simulink model "Aearial_Inspection_UAV_Simulation"  (R2023a)
settings: Solver=daessc  StartTime=0.0  StopTime=tf  MaxStep=0.1  MinStep=1e-30  RelTol=1e-4
values from neighbouring files (symbols this model uses):
  arm_start = 0    [InitScript.m]
  X = T*[x0;y0]    [line2circle.m]
undefined symbols (not defined in the file or in its folder): arm_end, DiscIntNeverNeededParam, F, is_gust_active, Light, MIL, Mode, Motor_data, params, Robotic_Arm_ASM_DataFile, Sensor_err, servo_specs, simple_env, stepper, Tm, wind_speed, xStack1, xStack2, Y, Z
libraries: sm_lib x399, nesl_utility x78, simulink x25, dspsrcs4 x16, simulink_extras x8, sharedtransform x7, aerolibwind2 x2, sharedutil x1
(part 4 of 12)

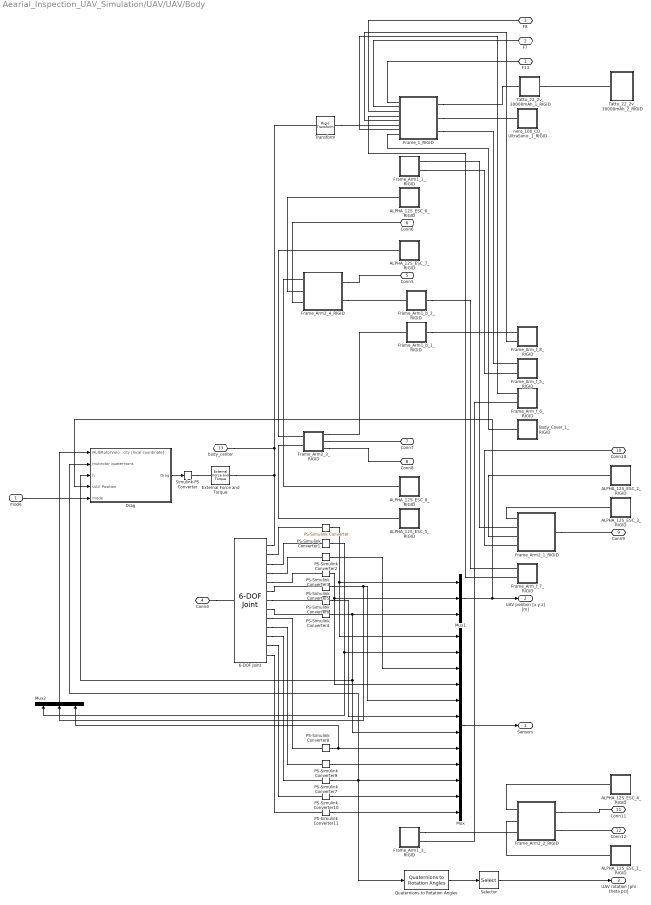
== system Aearial_Inspection_UAV_Simulation/UAV/UAV/Body ==
  mode : Inport
  " " : nesl_utility/PS-Simulink Converter  PhysicalDomain=network_engine_domain  SubClassName=ps_output  LeftPortType=input  RightPortType=output  PseudoPeriodic=off  Frequencies=[]  VectorFormat=1-D array  Unit=m  AffineConversion=off
  6-DOF Joint : sm_lib/Joints/6-DOF Joint  JointMode=Normal  SenseConstraintForce=off  SenseConstraintForceX=off  SenseConstraintForceY=off  SenseConstraintForceZ=off  SenseConstraintTorque=off  SenseConstraintTorqueX=off  SenseConstraintTorqueY=off  SenseConstraintTorqueZ=off  SenseTotalForce=off  SenseTotalForceX=off  SenseTotalForceY=off  SenseTotalForceZ=off  SenseTotalTorque=off  SenseTotalTorqueX=off  SenseTotalTorqueY=off  SenseTotalTorqueZ=off  CompositeWrenchDir=FollowerOnBase  CompositeWrenchFrame=BaseFrame  PxEquilibriumPosition=0  PxEquilibriumPositionUnits=m  PxSpringStiffness=0  PxSpringStiffnessUnits=N/m  PxDampingCoefficient=0  PxDampingCoefficientUnits=N/(m/s)  PxTorqueActuationMode=NoTorque  PxMotionActuationMode=ComputedMotion  PxSensePosition=on  PxSenseVelocity=on  PxSenseAcceleration=on  PxSenseTorqueForce=off  PxSenseLowerLimitTorqueForce=off  PxSenseUpperLimitTorqueForce=off  PxLowerLimitSpecify=off  PxLowerLimitBound=-1  PxLowerLimitBoundUnits=m  PxLowerLimitStiffness=1e6  PxLowerLimitStiffnessUnits=N/m  PxLowerLimitDamping=1e3  PxLowerLimitDampingUnits=N/(m/s)  PxLowerLimitTransitionRegionWidth=1e-4  PxLowerLimitTransitionRegionWidthUnits=m  PxUpperLimitSpecify=off  PxUpperLimitBound=1  PxUpperLimitBoundUnits=m  PxUpperLimitStiffness=1e6  PxUpperLimitStiffnessUnits=N/m  PxUpperLimitDamping=1e3  PxUpperLimitDampingUnits=N/(m/s)  PxUpperLimitTransitionRegionWidth=1e-4  PxUpperLimitTransitionRegionWidthUnits=m  PxPositionTargetSpecify=on  PxPositionTargetPriority=High  PxPositionTargetValue=params.pos0(1)  PxPositionTargetValueUnits=m  PxVelocityTargetSpecify=on  PxVelocityTargetPriority=High  PxVelocityTargetValue=params.vel0(1)  PxVelocityTargetValueUnits=m/s  PyEquilibriumPosition=0  PyEquilibriumPositionUnits=m  PySpringStiffness=0  PySpringStiffnessUnits=N/m  PyDampingCoefficient=0  PyDampingCoefficientUnits=N/(m/s)  PyTorqueActuationMode=NoTorque  PyMotionActuationMode=ComputedMotion  PySensePosition=on  PySenseVelocity=on  PySenseAcceleration=on  PySenseTorqueForce=off  PySenseLowerLimitTorqueForce=off  PySenseUpperLimitTorqueForce=off  PyLowerLimitSpecify=off  PyLowerLimitBound=-1  PyLowerLimitBoundUnits=m  PyLowerLimitStiffness=1e6  PyLowerLimitStiffnessUnits=N/m  PyLowerLimitDamping=1e3  PyLowerLimitDampingUnits=N/(m/s)  PyLowerLimitTransitionRegionWidth=1e-4  PyLowerLimitTransitionRegionWidthUnits=m  PyUpperLimitSpecify=off  PyUpperLimitBound=1  PyUpperLimitBoundUnits=m  PyUpperLimitStiffness=1e6  PyUpperLimitStiffnessUnits=N/m  PyUpperLimitDamping=1e3  PyUpperLimitDampingUnits=N/(m/s)  PyUpperLimitTransitionRegionWidth=1e-4  PyUpperLimitTransitionRegionWidthUnits=m  PyPositionTargetSpecify=on  PyPositionTargetPriority=High  PyPositionTargetValue=params.pos0(2)  PyPositionTargetValueUnits=m  PyVelocityTargetSpecify=on  PyVelocityTargetPriority=High  PyVelocityTargetValue=params.vel0(2)  PyVelocityTargetValueUnits=m/s  PzEquilibriumPosition=0  PzEquilibriumPositionUnits=m  PzSpringStiffness=0  PzSpringStiffnessUnits=N/m  PzDampingCoefficient=0  PzDampingCoefficientUnits=N/(m/s)  PzTorqueActuationMode=NoTorque  PzMotionActuationMode=ComputedMotion  PzSensePosition=on  PzSenseVelocity=on  PzSenseAcceleration=on  PzSenseTorqueForce=off  PzSenseLowerLimitTorqueForce=off  PzSenseUpperLimitTorqueForce=off  PzLowerLimitSpecify=off  PzLowerLimitBound=-1  PzLowerLimitBoundUnits=m  PzLowerLimitStiffness=1e6  PzLowerLimitStiffnessUnits=N/m  PzLowerLimitDamping=1e3  PzLowerLimitDampingUnits=N/(m/s)  PzLowerLimitTransitionRegionWidth=1e-4  PzLowerLimitTransitionRegionWidthUnits=m  PzUpperLimitSpecify=off  PzUpperLimitBound=1  PzUpperLimitBoundUnits=m  PzUpperLimitStiffness=1e6  PzUpperLimitStiffnessUnits=N/m  PzUpperLimitDamping=1e3  PzUpperLimitDampingUnits=N/(m/s)  PzUpperLimitTransitionRegionWidth=1e-4  PzUpperLimitTransitionRegionWidthUnits=m  PzPositionTargetSpecify=on  PzPositionTargetPriority=High  PzPositionTargetValue=params.pos0(3)  PzPositionTargetValueUnits=m  PzVelocityTargetSpecify=on  PzVelocityTargetPriority=High  PzVelocityTargetValue=params.vel0(3)  PzVelocityTargetValueUnits=m/s  SphEqPosRotationMethod=None  SphEqPosRotationAngleUnits=deg  SphEqPosRotationStandardAxis=+Z  SphEqPosRotationAngle=0.0  SphEqPosRotationArbitraryAxis=[0 0 1]  SphEqPosFollAlignAxisA=+X  SphEqPosBaseAlignAxisA=+Y  SphEqPosFollAlignAxisB=+Y  SphEqPosBaseAlignAxisB=+Z  SphEqPosRotationSequenceAxes=FollowerAxes  SphEqPosRotationSequence=XYX  SphEqPosRotationSequenceAngles=[0 0 0]  SphEqPosRotationSequenceAnglesUnits=deg  SphEqPosRotationMatrix=[1 0 0; 0 1 0; 0 0 1]  SphEqPosQuaternion=[1 0 0 0]  SphSpringStiffness=0  SphSpringStiffnessUnits=N*m/deg  SphDampingCoefficient=0  SphDampingCoefficientUnits=N*m/(deg/s)  SphActuateTorqueX=off  SphActuateTorqueY=off  SphActuateTorqueZ=off  SphActuateTorque=off  SphTorqueActuationMode=NoTorque  SphMotionActuationMode=ComputedMotion  SphActuationFrame=BaseFrame  SphSensePosition=on  SphSenseVelocityX=off  SphSenseVelocityY=off  SphSenseVelocityZ=off  SphSenseVelocity=on  SphSenseAccelerationX=off  SphSenseAccelerationY=off  SphSenseAccelerationZ=off  SphSenseAcceleration=on  SphSenseTorqueX=off  SphSenseTorqueY=off  SphSenseTorqueZ=off  SphSenseTorqueForce=off  SphSenseLowerLimitTorqueMag=off  SphSenseUpperLimitTorqueMag=off  SphSensingFrame=FollowerFrame  SphLowerLimitSpecify=off  SphLowerLimitBound=15  SphLowerLimitBoundUnits=deg  SphLowerLimitStiffness=1e4  SphLowerLimitStiffnessUnits=N*m/deg  SphLowerLimitDamping=10  SphLowerLimitDampingUnits=N*m/(deg/s)  SphLowerLimitTransitionRegionWidth=0.1  SphLowerLimitTransitionRegionWidthUnits=deg  SphUpperLimitSpecify=off  SphUpperLimitBound=45  SphUpperLimitBoundUnits=deg  SphUpperLimitStiffness=1e4  SphUpperLimitStiffnessUnits=N*m/deg  SphUpperLimitDamping=10  SphUpperLimitDampingUnits=N*m/(deg/s)  SphUpperLimitTransitionRegionWidth=0.1  SphUpperLimitTransitionRegionWidthUnits=deg  SphPositionTargetRotationMethod=RotationSequence  SphPositionTargetRotationAngleUnits=deg  SphPositionTargetRotationStandardAxis=+Z  SphPositionTargetRotationAngle=0.0  SphPositionTargetRotationArbitraryAxis=[0 0 1]  SphPositionTargetFollAlignAxisA=+X  SphPositionTargetBaseAlignAxisA=+Y  SphPositionTargetFollAlignAxisB=+Y  SphPositionTargetBaseAlignAxisB=+Z  SphPositionTargetRotationSequenceAxes=FollowerAxes  SphPositionTargetRotationSequence=XYZ  SphPositionTargetRotationSequenceAngles=params.Eul0  SphPositionTargetRotationSequenceAnglesUnits=deg  SphPositionTargetRotationMatrix=[1 0 0; 0 1 0; 0 0 1]  SphPositionTargetQuaternion=[1 0 0 0]  SphPositionTargetSpecify=on  SphPositionTargetPriority=High  SphVelocityTargetValue=params.Avel0  SphVelocityTargetValueUnits=deg/s  SphVelocityTargetSpecify=on  SphVelocityTargetPriority=High  SphVelocityTargetInFollowerFrame=on
  ALPHA_12S_ESC_1_RIGID : Subsystem
  ALPHA_12S_ESC_2_RIGID : Subsystem
  ALPHA_12S_ESC_3_RIGID : Subsystem
  ALPHA_12S_ESC_4_RIGID : Subsystem
  ALPHA_12S_ESC_5_RIGID : Subsystem
  ALPHA_12S_ESC_6_RIGID : Subsystem
  ALPHA_12S_ESC_7_RIGID : Subsystem
  ALPHA_12S_ESC_8_RIGID : Subsystem
  Body_Cover_1_RIGID : Subsystem
  Drag : Subsystem
  External Force and Torque : sm_lib/Forces and Torques/External Force and Torque  ForceResolutionFrame=AttachedFrame  EnableForceX=off  EnableForceY=off  EnableForceZ=off  EnableForce=on  TorqueResolutionFrame=AttachedFrame  EnableTorqueX=off  EnableTorqueY=off  EnableTorqueZ=off  EnableTorque=off
  Frame_1_RIGID : Subsystem
  Frame_Arm1_1_RIGID : Subsystem
  Frame_Arm1_3_RIGID : Subsystem
  Frame_Arm1_b_1_RIGID : Subsystem
  Frame_Arm1_b_2_RIGID : Subsystem
  Frame_Arm2_1_RIGID : Subsystem
  Frame_Arm2_2_RIGID : Subsystem
  Frame_Arm2_3_RIGID : Subsystem
  Frame_Arm2_4_RIGID : Subsystem
  Frame_Arm_f_5_RIGID : Subsystem
  Frame_Arm_f_6_RIGID : Subsystem
  Frame_Arm_f_7_RIGID : Subsystem
  Frame_Arm_f_8_RIGID : Subsystem
  Mux : Mux  Inputs=12
  Mux1 : Mux  Inputs=3
  Mux2 : Mux  Inputs=3
  PS-Simulink Converter1 : nesl_utility/PS-Simulink Converter  PhysicalDomain=network_engine_domain  SubClassName=ps_output  LeftPortType=input  RightPortType=output  PseudoPeriodic=off  Frequencies=[]  VectorFormat=1-D array  Unit=m/s  AffineConversion=off
  PS-Simulink Converter10 : nesl_utility/PS-Simulink Converter  PhysicalDomain=network_engine_domain  SubClassName=ps_output  LeftPortType=input  RightPortType=output  PseudoPeriodic=off  Frequencies=[]  VectorFormat=1-D array  Unit=rad/s  AffineConversion=off
  PS-Simulink Converter11 : nesl_utility/PS-Simulink Converter  PhysicalDomain=network_engine_domain  SubClassName=ps_output  LeftPortType=input  RightPortType=output  PseudoPeriodic=off  Frequencies=[]  VectorFormat=1-D array  Unit=rad/s^2  AffineConversion=off
  PS-Simulink Converter2 : nesl_utility/PS-Simulink Converter  PhysicalDomain=network_engine_domain  SubClassName=ps_output  LeftPortType=input  RightPortType=output  PseudoPeriodic=off  Frequencies=[]  VectorFormat=1-D array  Unit=m/s^2  AffineConversion=off
  PS-Simulink Converter3 : nesl_utility/PS-Simulink Converter  PhysicalDomain=network_engine_domain  SubClassName=ps_output  LeftPortType=input  RightPortType=output  PseudoPeriodic=off  Frequencies=[]  VectorFormat=1-D array  Unit=m  AffineConversion=off
  PS-Simulink Converter4 : nesl_utility/PS-Simulink Converter  PhysicalDomain=network_engine_domain  SubClassName=ps_output  LeftPortType=input  RightPortType=output  PseudoPeriodic=off  Frequencies=[]  VectorFormat=1-D array  Unit=m  AffineConversion=off
  PS-Simulink Converter5 : nesl_utility/PS-Simulink Converter  PhysicalDomain=network_engine_domain  SubClassName=ps_output  LeftPortType=input  RightPortType=output  PseudoPeriodic=off  Frequencies=[]  VectorFormat=1-D array  Unit=m/s  AffineConversion=off
  PS-Simulink Converter6 : nesl_utility/PS-Simulink Converter  PhysicalDomain=network_engine_domain  SubClassName=ps_output  LeftPortType=input  RightPortType=output  PseudoPeriodic=off  Frequencies=[]  VectorFormat=1-D array  Unit=m/s^2  AffineConversion=off
  PS-Simulink Converter7 : nesl_utility/PS-Simulink Converter  PhysicalDomain=network_engine_domain  SubClassName=ps_output  LeftPortType=input  RightPortType=output  PseudoPeriodic=off  Frequencies=[]  VectorFormat=1-D array  Unit=inherit  AffineConversion=off
  PS-Simulink Converter8 : nesl_utility/PS-Simulink Converter  PhysicalDomain=network_engine_domain  SubClassName=ps_output  LeftPortType=input  RightPortType=output  PseudoPeriodic=off  Frequencies=[]  VectorFormat=1-D array  Unit=m/s  AffineConversion=off
  PS-Simulink Converter9 : nesl_utility/PS-Simulink Converter  PhysicalDomain=network_engine_domain  SubClassName=ps_output  LeftPortType=input  RightPortType=output  PseudoPeriodic=off  Frequencies=[]  VectorFormat=1-D array  Unit=m/s^2  AffineConversion=off
  Quaternions to Rotation Angles : sharedtransform/Quaternions to Rotation Angles  rotationOrder=ZYX  aMode=aMode
  Selector : Selector  InputPortWidth=3  IndexOptions=Index vector (dialog)  Indices=[3 2 1]  OutputSizes=1
  Simulink-PS Converter : nesl_utility/Simulink-PS Converter  PhysicalDomain=network_engine_domain  SubClassName=ps_input  LeftPortType=input  RightPortType=output  PseudoPeriodic=off  Frequencies=[]  NoiseDistribution=none  NoiseParameters=[]  Unit=N  AffineConversion=off  FilteringAndDerivatives=provide  SimscapeFilterOrder=1  InputFilterTimeConstant=0.001  UdotUserProvided=0
  Tattu_22_2v_30000mAh_1_RIGID : Subsystem
  Tattu_22_2v_30000mAh_2_RIGID : Subsystem
  Transform : sm_lib/Frames and Transforms/Rigid Transform  TranslationMethod=Cartesian  TranslationStandardOffset=0  TranslationStandardOffsetUnits=mm  TranslationStandardAxis=+Z  TranslationCartesianOffset=[0.2 0 0]  TranslationCartesianOffsetUnits=mm  TranslationROffset=0  TranslationROffsetUnits=m  TranslationZOffset=0  TranslationZOffsetUnits=m  TranslationThetaOffset=0  TranslationThetaOffsetUnits=deg  RotationMethod=AlignedAxes  RotationAngleUnits=rad  RotationStandardAxis=+Z  RotationAngle=smiData.RigidTransform(347).angle  RotationArbitraryAxis=smiData.RigidTransform(347).axis  FollAlignAxisA=+X  BaseAlignAxisA=+Y  FollAlignAxisB=+Y  BaseAlignAxisB=-Z  RotationSequenceAxes=FollowerAxes  RotationSequence=XYX  RotationSequenceAngles=[0 0 0]  RotationSequenceAnglesUnits=deg  RotationMatrix=[1 0 0; 0 1 0; 0 0 1]  Quaternion=[1 0 0 0]
  nero_100_CD_UltraSonic_1_RIGID : Subsystem
  F13 : PMIOPort  Side=Left
  F7 : PMIOPort  Port=2  Side=Left
  F8 : PMIOPort  Port=3  Side=Left
  Conn4 : PMIOPort  Port=4  Side=Left
  Conn5 : PMIOPort  Port=5  Side=Right
  Conn6 : PMIOPort  Port=6  Side=Right
  Conn7 : PMIOPort  Port=7  Side=Right
  Conn8 : PMIOPort  Port=8  Side=Right
  Conn9 : PMIOPort  Port=9  Side=Right
  Conn10 : PMIOPort  Port=10  Side=Right
  Conn11 : PMIOPort  Port=11  Side=Right
  Conn12 : PMIOPort  Port=12  Side=Right
  body_center : PMIOPort  Port=13  Side=Left
  Sensors : Outport
  UAV position [x y z] [m] : Outport  Port=2
  UAV rotation [phi theta psi] : Outport  Port=3
  wires:
  PS-Simulink Converter8/1 -> Mux2/3, Mux/8
  Mux/1 -> Sensors/1
  PS-Simulink Converter10/1 -> Mux/11
  Quaternions to Rotation Angles/1 -> Selector/1
  Mux1/1 -> Drag/4(UAV Position), UAV position [x y z] [m]/1
  PS-Simulink Converter11/1 -> Mux/12
  PS-Simulink Converter9/1 -> Mux/9
  PS-Simulink Converter6/1 -> Mux/6
  PS-Simulink Converter5/1 -> Mux2/2, Mux/5
  PS-Simulink Converter2/1 -> Mux/3
  PS-Simulink Converter1/1 -> Mux2/1, Mux/2
  PS-Simulink Converter7/1 -> Quaternions to Rotation Angles/1, Drag/2(mutirotor quaternions), Mux/10
  PS-Simulink Converter4/1 -> Drag/3(h), Mux/7, Mux1/3
  PS-Simulink Converter3/1 -> Mux1/2, Mux/4
  " "/1 -> Mux1/1, Mux/1
  Mux2/1 -> Drag/1(MultiRotorVelocity [local coordinate])
  Drag/1(Drag) -> Simulink-PS Converter/1
  mode/1 -> Drag/5(mode)
  Selector/1 -> UAV rotation [phi theta psi]/1
  connections:
  6-DOF Joint/RConn11 -- PS-Simulink Converter7/LConn1
  Transform/RConn1 -- Frame_1_RIGID/LConn6
  ALPHA_12S_ESC_5_RIGID/LConn1 -- Frame_Arm2_3_RIGID/LConn2
  Frame_1_RIGID/LConn3 -- F8/RConn1
  6-DOF Joint/RConn6 -- PS-Simulink Converter5/LConn1
  Frame_Arm2_2_RIGID/RConn2 -- Conn12/RConn1
  ALPHA_12S_ESC_3_RIGID/LConn1 -- Frame_Arm2_1_RIGID/LConn1
  Frame_1_RIGID/RConn2 -- nero_100_CD_UltraSonic_1_RIGID/LConn1
  6-DOF Joint/RConn13 -- PS-Simulink Converter11/LConn1
  ALPHA_12S_ESC_6_RIGID/LConn1 -- Frame_Arm2_4_RIGID/LConn2
  Frame_1_RIGID/RConn1 -- Tattu_22_2v_30000mAh_1_RIGID/LConn1
  6-DOF Joint/RConn12 -- PS-Simulink Converter10/LConn1
  Frame_1_RIGID/LConn7 -- Frame_Arm_f_6_RIGID/LConn1
  6-DOF Joint/RConn10 -- PS-Simulink Converter9/LConn1
  6-DOF Joint/RConn9 -- PS-Simulink Converter8/LConn1
  Frame_1_RIGID/LConn4 -- Frame_Arm_f_7_RIGID/LConn2
  6-DOF Joint/RConn7 -- PS-Simulink Converter6/LConn1
  Frame_1_RIGID/LConn5 -- Frame_Arm_f_8_RIGID/LConn2
  6-DOF Joint/RConn8 -- PS-Simulink Converter4/LConn1
  6-DOF Joint/RConn5 -- PS-Simulink Converter3/LConn1
  6-DOF Joint/RConn4 -- PS-Simulink Converter2/LConn1
  6-DOF Joint/RConn3 -- PS-Simulink Converter1/LConn1
  6-DOF Joint/RConn2 -- " "/LConn1
  6-DOF Joint/RConn1 -- External Force and Torque/RConn1 -- body_center/RConn1 -- Transform/LConn1
  ALPHA_12S_ESC_4_RIGID/LConn1 -- Frame_Arm2_2_RIGID/LConn1
  F13/RConn1 -- Frame_1_RIGID/LConn1
  Conn4/RConn1 -- 6-DOF Joint/LConn1
  Frame_Arm1_3_RIGID/RConn2 -- Frame_Arm_f_6_RIGID/LConn2
  Frame_Arm2_1_RIGID/LConn4 -- Conn10/RConn1
  Tattu_22_2v_30000mAh_1_RIGID/RConn1 -- Tattu_22_2v_30000mAh_2_RIGID/LConn1
  F7/RConn1 -- Frame_1_RIGID/LConn2
  Conn6/RConn1 -- Frame_Arm2_4_RIGID/LConn3
  Frame_Arm1_b_2_RIGID/RConn1 -- Frame_Arm_f_7_RIGID/LConn1
  ALPHA_12S_ESC_2_RIGID/LConn1 -- Frame_Arm2_1_RIGID/LConn3
  Frame_Arm2_2_RIGID/RConn1 -- Conn11/RConn1
  Frame_Arm1_1_RIGID/RConn2 -- Frame_Arm_f_5_RIGID/LConn2
  Frame_1_RIGID/RConn3 -- Frame_Arm_f_5_RIGID/LConn1
  ALPHA_12S_ESC_1_RIGID/LConn1 -- Frame_Arm2_2_RIGID/LConn2
  ALPHA_12S_ESC_8_RIGID/LConn1 -- Frame_Arm2_4_RIGID/LConn1
  Body_Cover_1_RIGID/LConn1 -- Frame_1_RIGID/LConn8
  Frame_Arm2_3_RIGID/RConn1 -- Frame_Arm1_b_1_RIGID/LConn1
  Frame_Arm2_1_RIGID/RConn1 -- Conn9/RConn1
  Frame_Arm2_4_RIGID/RConn2 -- Frame_Arm1_b_2_RIGID/LConn1
  Frame_Arm2_3_RIGID/RConn3 -- Conn8/RConn1
  Frame_Arm1_3_RIGID/RConn1 -- Frame_Arm2_2_RIGID/LConn3
  Frame_Arm2_4_RIGID/RConn1 -- Conn5/RConn1
  Frame_Arm2_3_RIGID/RConn2 -- Conn7/RConn1
  ALPHA_12S_ESC_7_RIGID/LConn1 -- Frame_Arm2_3_RIGID/LConn1
  Frame_Arm1_b_1_RIGID/RConn1 -- Frame_Arm_f_8_RIGID/LConn1
  Frame_Arm1_1_RIGID/RConn1 -- Frame_Arm2_1_RIGID/LConn2
  Simulink-PS Converter/RConn1 -- External Force and Torque/LConn1

== system Aearial_Inspection_UAV_Simulation/UAV/UAV/Device ==
  Device_1_RIGID : Subsystem
  Device_Box_1_RIGID : Subsystem
  F : PMIOPort  Side=Left
  connections:
  Device_1_RIGID/LConn1 -- Device_Box_1_RIGID/LConn1
  Device_Box_1_RIGID/LConn2 -- F/RConn1

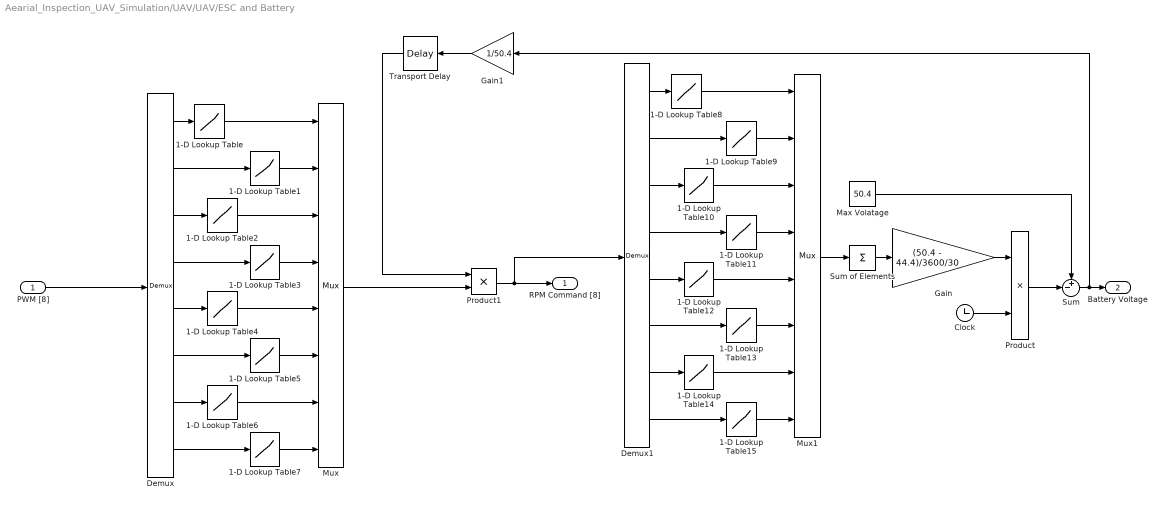
== system Aearial_Inspection_UAV_Simulation/UAV/UAV/ESC and Battery ==
  PWM [8] : Inport
  1-D Lookup Table{,1..7} (8 alike) : Lookup_n-D  NumberOfTableDimensions=1  BreakpointsForDimension1=[0;Motor_data.Throttle]  Table=[0;Motor_data.RPM]  InternalRulePriority=Speed  RndMeth=Simplest
  1-D Lookup Table{8..15} (8 alike) : Lookup_n-D  NumberOfTableDimensions=1  BreakpointsForDimension1=[0;Motor_data.RPM]  Table=[0;Motor_data.Current]  InterpMethod=Cubic spline  ExtrapMethod=Cubic spline  InternalRulePriority=Speed  RndMeth=Simplest
  Clock : Clock
  Demux : Demux  Outputs=8
  Demux1 : Demux  Outputs=8
  Gain : Gain  Gain=(50.4 - 44.4)/3600/30
  Gain1 : Gain  Gain=1/50.4
  Max Volatage : Constant  Value=50.4
  Mux : Mux  Inputs=8
  Mux1 : Mux  Inputs=8
  Product : Product
  Product1 : Product
  Sum : Sum  Inputs=+-|
  Sum of Elements : Sum  Inputs=+
  Transport Delay : TransportDelay  DelayTime=0.001
  RPM Command [8] : Outport
  Battery Voltage : Outport  Port=2
  wires:
  PWM [8]/1 -> Demux/1
  Demux/1 -> 1-D Lookup Table/1
  Demux/2 -> 1-D Lookup Table1/1
  Demux/3 -> 1-D Lookup Table2/1
  Demux/4 -> 1-D Lookup Table3/1
  Demux/5 -> 1-D Lookup Table4/1
  Demux/6 -> 1-D Lookup Table5/1
  Demux/7 -> 1-D Lookup Table6/1
  Demux/8 -> 1-D Lookup Table7/1
  1-D Lookup Table7/1 -> Mux/8
  1-D Lookup Table5/1 -> Mux/6
  1-D Lookup Table3/1 -> Mux/4
  1-D Lookup Table1/1 -> Mux/2
  1-D Lookup Table6/1 -> Mux/7
  1-D Lookup Table4/1 -> Mux/5
  1-D Lookup Table2/1 -> Mux/3
  1-D Lookup Table/1 -> Mux/1
  1-D Lookup Table8/1 -> Mux1/1
  1-D Lookup Table10/1 -> Mux1/3
  1-D Lookup Table12/1 -> Mux1/5
  1-D Lookup Table14/1 -> Mux1/7
  1-D Lookup Table9/1 -> Mux1/2
  1-D Lookup Table11/1 -> Mux1/4
  1-D Lookup Table13/1 -> Mux1/6
  1-D Lookup Table15/1 -> Mux1/8
  Demux1/8 -> 1-D Lookup Table15/1
  Demux1/7 -> 1-D Lookup Table14/1
  Demux1/6 -> 1-D Lookup Table13/1
  Demux1/5 -> 1-D Lookup Table12/1
  Demux1/4 -> 1-D Lookup Table11/1
  Demux1/3 -> 1-D Lookup Table10/1
  Demux1/2 -> 1-D Lookup Table9/1
  Demux1/1 -> 1-D Lookup Table8/1
  Mux1/1 -> Sum of Elements/1
  Sum of Elements/1 -> Gain/1
  Product/1 -> Sum/2
  Gain/1 -> Product/1
  Clock/1 -> Product/2
  Max Volatage/1 -> Sum/1
  Sum/1 -> Gain1/1, Battery Voltage/1
  Product1/1 -> RPM Command [8]/1, Demux1/1
  Gain1/1 -> Transport Delay/1
  Transport Delay/1 -> Product1/1
  Mux/1 -> Product1/2

== system Aearial_Inspection_UAV_Simulation/UAV/UAV/Landing Gear ==
  Front_lastic_1_RIGID : Subsystem
  Front_lastic_2_RIGID : Subsystem
  Landing_Gear_5_RIGID : Subsystem
  Rear_lastic_1_RIGID : Subsystem
  Rear_lastic_2_RIGID : Subsystem
  F : PMIOPort  Side=Left
  connections:
  Rear_lastic_2_RIGID/LConn1 -- Landing_Gear_5_RIGID/RConn3
  Front_lastic_2_RIGID/LConn1 -- Landing_Gear_5_RIGID/RConn1
  Front_lastic_1_RIGID/LConn1 -- Landing_Gear_5_RIGID/RConn2
  Landing_Gear_5_RIGID/RConn4 -- Rear_lastic_1_RIGID/LConn1
  F/RConn1 -- Landing_Gear_5_RIGID/LConn1

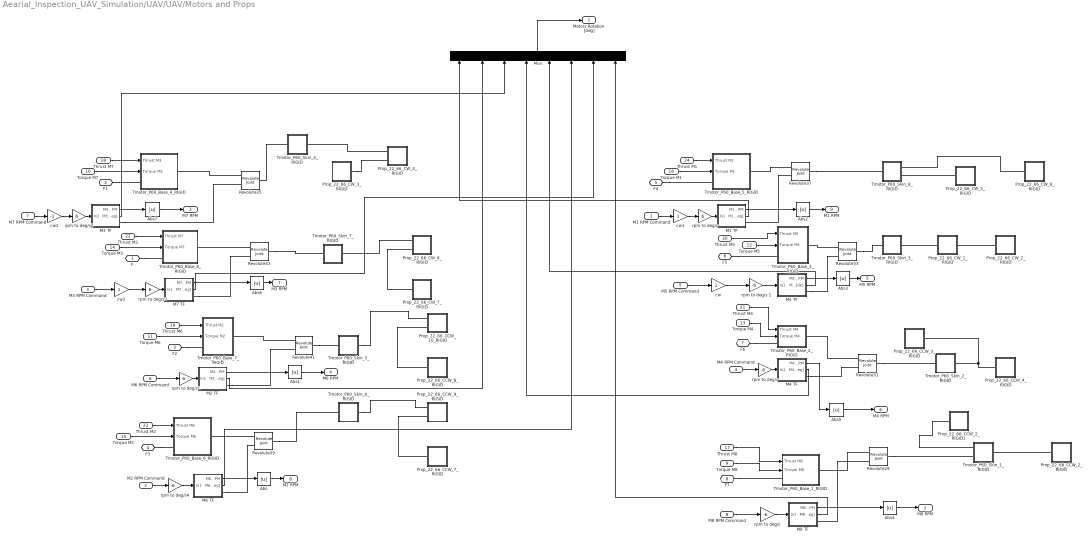
== system Aearial_Inspection_UAV_Simulation/UAV/UAV/Motors and Props ==
  M1 RPM Command : Inport
  M2 RPM Command : Inport  Port=2
  M3 RPM Command : Inport  Port=3
  M4 RPM Command : Inport  Port=4
  M5 RPM Command : Inport  Port=5
  M6 RPM Command : Inport  Port=6
  M7 RPM Command : Inport  Port=7
  M8 RPM Command : Inport  Port=8
  Torque M8 : Inport  Port=9
  Torque M7 : Inport  Port=10
  Torque M6 : Inport  Port=11
  Torque M5 : Inport  Port=12
  Torque M4 : Inport  Port=13
  Torque M3 : Inport  Port=14
  Torque M2 : Inport  Port=15
  Torque M1 : Inport  Port=16
  Thrust M8 : Inport  Port=17
  Thrust M7 : Inport  Port=18
  Thrust M6 : Inport  Port=19
  Thrust M5 : Inport  Port=20
  Thrust M4 : Inport  Port=21
  Thrust M3 : Inport  Port=22
  Thrust M2 : Inport  Port=23
  Thrust M1 : Inport  Port=24
  Abs{,1..7} (8 alike) : Abs  SaturateOnIntegerOverflow=off
  M1 TF : Subsystem
  M2 TF : Subsystem
  M3 TF : Subsystem
  M4 TF : Subsystem
  M5 TF : Subsystem
  M6 TF : Subsystem
  M7 TF : Subsystem
  M8 TF : Subsystem
  Mux : Mux  Inputs=8
  Prop_22_66_CCW_10_RIGID : Subsystem
  Prop_22_66_CCW_2_RIGID : Subsystem
  Prop_22_66_CCW_2_RIGID1 : Subsystem
  Prop_22_66_CCW_3_RIGID : Subsystem
  Prop_22_66_CCW_4_RIGID : Subsystem
  Prop_22_66_CCW_7_RIGID : Subsystem
  Prop_22_66_CCW_8_RIGID : Subsystem
  Prop_22_66_CCW_9_RIGID : Subsystem
  Prop_22_66_CW_1_RIGID : Subsystem
  Prop_22_66_CW_2_RIGID : Subsystem
  Prop_22_66_CW_3_RIGID : Subsystem
  Prop_22_66_CW_4_RIGID : Subsystem
  Prop_22_66_CW_5_RIGID : Subsystem
  Prop_22_66_CW_6_RIGID : Subsystem
  Prop_22_66_CW_7_RIGID : Subsystem
  Prop_22_66_CW_8_RIGID : Subsystem
  Revolute29 : sm_lib/Joints/Revolute Joint  JointMode=Normal  SenseConstraintForce=off  SenseConstraintForceX=off  SenseConstraintForceY=off  SenseConstraintForceZ=off  SenseConstraintTorque=off  SenseConstraintTorqueX=off  SenseConstraintTorqueY=off  SenseConstraintTorqueZ=off  SenseTotalForce=off  SenseTotalForceX=off  SenseTotalForceY=off  SenseTotalForceZ=off  SenseTotalTorque=off  SenseTotalTorqueX=off  SenseTotalTorqueY=off  SenseTotalTorqueZ=off  CompositeWrenchDir=FollowerOnBase  CompositeWrenchFrame=BaseFrame  EquilibriumPosition=0  EquilibriumPositionUnits=deg  SpringStiffness=0  SpringStiffnessUnits=N*m/deg  DampingCoefficient=0  DampingCoefficientUnits=N*m/(deg/s)  TorqueActuationMode=ComputedTorque  MotionActuationMode=InputMotion  SensePosition=off  SenseVelocity=off  SenseAcceleration=off  SenseTorqueForce=off  SenseLowerLimitTorqueForce=off  SenseUpperLimitTorqueForce=off  LowerLimitSpecify=off  LowerLimitBound=-90  LowerLimitBoundUnits=deg  LowerLimitStiffness=1e4  LowerLimitStiffnessUnits=N*m/deg  LowerLimitDamping=10  LowerLimitDampingUnits=N*m/(deg/s)  LowerLimitTransitionRegionWidth=0.1  LowerLimitTransitionRegionWidthUnits=deg  UpperLimitSpecify=off  UpperLimitBound=90  UpperLimitBoundUnits=deg  UpperLimitStiffness=1e4  UpperLimitStiffnessUnits=N*m/deg  UpperLimitDamping=10  UpperLimitDampingUnits=N*m/(deg/s)  UpperLimitTransitionRegionWidth=0.1  UpperLimitTransitionRegionWidthUnits=deg  PositionTargetSpecify=on  PositionTargetPriority=Low  PositionTargetValue=smiData.RevoluteJoint(30).Rz.Pos  PositionTargetValueUnits=deg  VelocityTargetSpecify=off  VelocityTargetPriority=High  VelocityTargetValue=0  VelocityTargetValueUnits=deg/s
  Revolute31 : sm_lib/Joints/Revolute Joint  JointMode=Normal  SenseConstraintForce=off  SenseConstraintForceX=off  SenseConstraintForceY=off  SenseConstraintForceZ=off  SenseConstraintTorque=off  SenseConstraintTorqueX=off  SenseConstraintTorqueY=off  SenseConstraintTorqueZ=off  SenseTotalForce=off  SenseTotalForceX=off  SenseTotalForceY=off  SenseTotalForceZ=off  SenseTotalTorque=off  SenseTotalTorqueX=off  SenseTotalTorqueY=off  SenseTotalTorqueZ=off  CompositeWrenchDir=FollowerOnBase  CompositeWrenchFrame=BaseFrame  EquilibriumPosition=0  EquilibriumPositionUnits=deg  SpringStiffness=0  SpringStiffnessUnits=N*m/deg  DampingCoefficient=0  DampingCoefficientUnits=N*m/(deg/s)  TorqueActuationMode=ComputedTorque  MotionActuationMode=InputMotion  SensePosition=off  SenseVelocity=off  SenseAcceleration=off  SenseTorqueForce=off  SenseLowerLimitTorqueForce=off  SenseUpperLimitTorqueForce=off  LowerLimitSpecify=off  LowerLimitBound=-90  LowerLimitBoundUnits=deg  LowerLimitStiffness=1e4  LowerLimitStiffnessUnits=N*m/deg  LowerLimitDamping=10  LowerLimitDampingUnits=N*m/(deg/s)  LowerLimitTransitionRegionWidth=0.1  LowerLimitTransitionRegionWidthUnits=deg  UpperLimitSpecify=off  UpperLimitBound=90  UpperLimitBoundUnits=deg  UpperLimitStiffness=1e4  UpperLimitStiffnessUnits=N*m/deg  UpperLimitDamping=10  UpperLimitDampingUnits=N*m/(deg/s)  UpperLimitTransitionRegionWidth=0.1  UpperLimitTransitionRegionWidthUnits=deg  PositionTargetSpecify=on  PositionTargetPriority=Low  PositionTargetValue=smiData.RevoluteJoint(32).Rz.Pos  PositionTargetValueUnits=deg  VelocityTargetSpecify=off  VelocityTargetPriority=High  VelocityTargetValue=0  VelocityTargetValueUnits=deg/s
  Revolute33 : sm_lib/Joints/Revolute Joint  JointMode=Normal  SenseConstraintForce=off  SenseConstraintForceX=off  SenseConstraintForceY=off  SenseConstraintForceZ=off  SenseConstraintTorque=off  SenseConstraintTorqueX=off  SenseConstraintTorqueY=off  SenseConstraintTorqueZ=off  SenseTotalForce=off  SenseTotalForceX=off  SenseTotalForceY=off  SenseTotalForceZ=off  SenseTotalTorque=off  SenseTotalTorqueX=off  SenseTotalTorqueY=off  SenseTotalTorqueZ=off  CompositeWrenchDir=FollowerOnBase  CompositeWrenchFrame=BaseFrame  EquilibriumPosition=0  EquilibriumPositionUnits=deg  SpringStiffness=0  SpringStiffnessUnits=N*m/deg  DampingCoefficient=0  DampingCoefficientUnits=N*m/(deg/s)  TorqueActuationMode=ComputedTorque  MotionActuationMode=InputMotion  SensePosition=off  SenseVelocity=off  SenseAcceleration=off  SenseTorqueForce=off  SenseLowerLimitTorqueForce=off  SenseUpperLimitTorqueForce=off  LowerLimitSpecify=off  LowerLimitBound=-90  LowerLimitBoundUnits=deg  LowerLimitStiffness=1e4  LowerLimitStiffnessUnits=N*m/deg  LowerLimitDamping=10  LowerLimitDampingUnits=N*m/(deg/s)  LowerLimitTransitionRegionWidth=0.1  LowerLimitTransitionRegionWidthUnits=deg  UpperLimitSpecify=off  UpperLimitBound=90  UpperLimitBoundUnits=deg  UpperLimitStiffness=1e4  UpperLimitStiffnessUnits=N*m/deg  UpperLimitDamping=10  UpperLimitDampingUnits=N*m/(deg/s)  UpperLimitTransitionRegionWidth=0.1  UpperLimitTransitionRegionWidthUnits=deg  PositionTargetSpecify=on  PositionTargetPriority=Low  PositionTargetValue=smiData.RevoluteJoint(34).Rz.Pos  PositionTargetValueUnits=deg  VelocityTargetSpecify=off  VelocityTargetPriority=High  VelocityTargetValue=0  VelocityTargetValueUnits=deg/s
  Revolute35 : sm_lib/Joints/Revolute Joint  JointMode=Normal  SenseConstraintForce=off  SenseConstraintForceX=off  SenseConstraintForceY=off  SenseConstraintForceZ=off  SenseConstraintTorque=off  SenseConstraintTorqueX=off  SenseConstraintTorqueY=off  SenseConstraintTorqueZ=off  SenseTotalForce=off  SenseTotalForceX=off  SenseTotalForceY=off  SenseTotalForceZ=off  SenseTotalTorque=off  SenseTotalTorqueX=off  SenseTotalTorqueY=off  SenseTotalTorqueZ=off  CompositeWrenchDir=FollowerOnBase  CompositeWrenchFrame=BaseFrame  EquilibriumPosition=0  EquilibriumPositionUnits=deg  SpringStiffness=0  SpringStiffnessUnits=N*m/deg  DampingCoefficient=0  DampingCoefficientUnits=N*m/(deg/s)  TorqueActuationMode=ComputedTorque  MotionActuationMode=InputMotion  SensePosition=off  SenseVelocity=off  SenseAcceleration=off  SenseTorqueForce=off  SenseLowerLimitTorqueForce=off  SenseUpperLimitTorqueForce=off  LowerLimitSpecify=off  LowerLimitBound=-90  LowerLimitBoundUnits=deg  LowerLimitStiffness=1e4  LowerLimitStiffnessUnits=N*m/deg  LowerLimitDamping=10  LowerLimitDampingUnits=N*m/(deg/s)  LowerLimitTransitionRegionWidth=0.1  LowerLimitTransitionRegionWidthUnits=deg  UpperLimitSpecify=off  UpperLimitBound=90  UpperLimitBoundUnits=deg  UpperLimitStiffness=1e4  UpperLimitStiffnessUnits=N*m/deg  UpperLimitDamping=10  UpperLimitDampingUnits=N*m/(deg/s)  UpperLimitTransitionRegionWidth=0.1  UpperLimitTransitionRegionWidthUnits=deg  PositionTargetSpecify=on  PositionTargetPriority=Low  PositionTargetValue=smiData.RevoluteJoint(36).Rz.Pos  PositionTargetValueUnits=deg  VelocityTargetSpecify=off  VelocityTargetPriority=High  VelocityTargetValue=0  VelocityTargetValueUnits=deg/s
  Revolute37 : sm_lib/Joints/Revolute Joint  JointMode=Normal  SenseConstraintForce=off  SenseConstraintForceX=off  SenseConstraintForceY=off  SenseConstraintForceZ=off  SenseConstraintTorque=off  SenseConstraintTorqueX=off  SenseConstraintTorqueY=off  SenseConstraintTorqueZ=off  SenseTotalForce=off  SenseTotalForceX=off  SenseTotalForceY=off  SenseTotalForceZ=off  SenseTotalTorque=off  SenseTotalTorqueX=off  SenseTotalTorqueY=off  SenseTotalTorqueZ=off  CompositeWrenchDir=FollowerOnBase  CompositeWrenchFrame=BaseFrame  EquilibriumPosition=0  EquilibriumPositionUnits=deg  SpringStiffness=0  SpringStiffnessUnits=N*m/deg  DampingCoefficient=0  DampingCoefficientUnits=N*m/(deg/s)  TorqueActuationMode=ComputedTorque  MotionActuationMode=InputMotion  SensePosition=off  SenseVelocity=off  SenseAcceleration=off  SenseTorqueForce=off  SenseLowerLimitTorqueForce=off  SenseUpperLimitTorqueForce=off  LowerLimitSpecify=off  LowerLimitBound=-90  LowerLimitBoundUnits=deg  LowerLimitStiffness=1e4  LowerLimitStiffnessUnits=N*m/deg  LowerLimitDamping=10  LowerLimitDampingUnits=N*m/(deg/s)  LowerLimitTransitionRegionWidth=0.1  LowerLimitTransitionRegionWidthUnits=deg  UpperLimitSpecify=off  UpperLimitBound=90  UpperLimitBoundUnits=deg  UpperLimitStiffness=1e4  UpperLimitStiffnessUnits=N*m/deg  UpperLimitDamping=10  UpperLimitDampingUnits=N*m/(deg/s)  UpperLimitTransitionRegionWidth=0.1  UpperLimitTransitionRegionWidthUnits=deg  PositionTargetSpecify=on  PositionTargetPriority=Low  PositionTargetValue=smiData.RevoluteJoint(38).Rz.Pos  PositionTargetValueUnits=deg  VelocityTargetSpecify=off  VelocityTargetPriority=High  VelocityTargetValue=0  VelocityTargetValueUnits=deg/s
  Revolute39 : sm_lib/Joints/Revolute Joint  JointMode=Normal  SenseConstraintForce=off  SenseConstraintForceX=off  SenseConstraintForceY=off  SenseConstraintForceZ=off  SenseConstraintTorque=off  SenseConstraintTorqueX=off  SenseConstraintTorqueY=off  SenseConstraintTorqueZ=off  SenseTotalForce=off  SenseTotalForceX=off  SenseTotalForceY=off  SenseTotalForceZ=off  SenseTotalTorque=off  SenseTotalTorqueX=off  SenseTotalTorqueY=off  SenseTotalTorqueZ=off  CompositeWrenchDir=FollowerOnBase  CompositeWrenchFrame=BaseFrame  EquilibriumPosition=0  EquilibriumPositionUnits=deg  SpringStiffness=0  SpringStiffnessUnits=N*m/deg  DampingCoefficient=0  DampingCoefficientUnits=N*m/(deg/s)  TorqueActuationMode=ComputedTorque  MotionActuationMode=InputMotion  SensePosition=off  SenseVelocity=off  SenseAcceleration=off  SenseTorqueForce=off  SenseLowerLimitTorqueForce=off  SenseUpperLimitTorqueForce=off  LowerLimitSpecify=off  LowerLimitBound=-90  LowerLimitBoundUnits=deg  LowerLimitStiffness=1e4  LowerLimitStiffnessUnits=N*m/deg  LowerLimitDamping=10  LowerLimitDampingUnits=N*m/(deg/s)  LowerLimitTransitionRegionWidth=0.1  LowerLimitTransitionRegionWidthUnits=deg  UpperLimitSpecify=off  UpperLimitBound=90  UpperLimitBoundUnits=deg  UpperLimitStiffness=1e4  UpperLimitStiffnessUnits=N*m/deg  UpperLimitDamping=10  UpperLimitDampingUnits=N*m/(deg/s)  UpperLimitTransitionRegionWidth=0.1  UpperLimitTransitionRegionWidthUnits=deg  PositionTargetSpecify=on  PositionTargetPriority=Low  PositionTargetValue=smiData.RevoluteJoint(40).Rz.Pos  PositionTargetValueUnits=deg  VelocityTargetSpecify=off  VelocityTargetPriority=High  VelocityTargetValue=0  VelocityTargetValueUnits=deg/s
  Revolute41 : sm_lib/Joints/Revolute Joint  JointMode=Normal  SenseConstraintForce=off  SenseConstraintForceX=off  SenseConstraintForceY=off  SenseConstraintForceZ=off  SenseConstraintTorque=off  SenseConstraintTorqueX=off  SenseConstraintTorqueY=off  SenseConstraintTorqueZ=off  SenseTotalForce=off  SenseTotalForceX=off  SenseTotalForceY=off  SenseTotalForceZ=off  SenseTotalTorque=off  SenseTotalTorqueX=off  SenseTotalTorqueY=off  SenseTotalTorqueZ=off  CompositeWrenchDir=FollowerOnBase  CompositeWrenchFrame=BaseFrame  EquilibriumPosition=0  EquilibriumPositionUnits=deg  SpringStiffness=0  SpringStiffnessUnits=N*m/deg  DampingCoefficient=0  DampingCoefficientUnits=N*m/(deg/s)  TorqueActuationMode=ComputedTorque  MotionActuationMode=InputMotion  SensePosition=off  SenseVelocity=off  SenseAcceleration=off  SenseTorqueForce=off  SenseLowerLimitTorqueForce=off  SenseUpperLimitTorqueForce=off  LowerLimitSpecify=off  LowerLimitBound=-90  LowerLimitBoundUnits=deg  LowerLimitStiffness=1e4  LowerLimitStiffnessUnits=N*m/deg  LowerLimitDamping=10  LowerLimitDampingUnits=N*m/(deg/s)  LowerLimitTransitionRegionWidth=0.1  LowerLimitTransitionRegionWidthUnits=deg  UpperLimitSpecify=off  UpperLimitBound=90  UpperLimitBoundUnits=deg  UpperLimitStiffness=1e4  UpperLimitStiffnessUnits=N*m/deg  UpperLimitDamping=10  UpperLimitDampingUnits=N*m/(deg/s)  UpperLimitTransitionRegionWidth=0.1  UpperLimitTransitionRegionWidthUnits=deg  PositionTargetSpecify=off  PositionTargetPriority=Low  PositionTargetValue=smiData.RevoluteJoint(42).Rz.Pos  PositionTargetValueUnits=deg  VelocityTargetSpecify=off  VelocityTargetPriority=High  VelocityTargetValue=100  VelocityTargetValueUnits=deg/s
  Revolute43 : sm_lib/Joints/Revolute Joint  JointMode=Normal  SenseConstraintForce=off  SenseConstraintForceX=off  SenseConstraintForceY=off  SenseConstraintForceZ=off  SenseConstraintTorque=off  SenseConstraintTorqueX=off  SenseConstraintTorqueY=off  SenseConstraintTorqueZ=off  SenseTotalForce=off  SenseTotalForceX=off  SenseTotalForceY=off  SenseTotalForceZ=off  SenseTotalTorque=off  SenseTotalTorqueX=off  SenseTotalTorqueY=off  SenseTotalTorqueZ=off  CompositeWrenchDir=FollowerOnBase  CompositeWrenchFrame=BaseFrame  EquilibriumPosition=0  EquilibriumPositionUnits=deg  SpringStiffness=0  SpringStiffnessUnits=N*m/deg  DampingCoefficient=0  DampingCoefficientUnits=N*m/(deg/s)  TorqueActuationMode=ComputedTorque  MotionActuationMode=InputMotion  SensePosition=off  SenseVelocity=off  SenseAcceleration=off  SenseTorqueForce=off  SenseLowerLimitTorqueForce=off  SenseUpperLimitTorqueForce=off  LowerLimitSpecify=off  LowerLimitBound=-90  LowerLimitBoundUnits=deg  LowerLimitStiffness=1e4  LowerLimitStiffnessUnits=N*m/deg  LowerLimitDamping=10  LowerLimitDampingUnits=N*m/(deg/s)  LowerLimitTransitionRegionWidth=0.1  LowerLimitTransitionRegionWidthUnits=deg  UpperLimitSpecify=off  UpperLimitBound=90  UpperLimitBoundUnits=deg  UpperLimitStiffness=1e4  UpperLimitStiffnessUnits=N*m/deg  UpperLimitDamping=10  UpperLimitDampingUnits=N*m/(deg/s)  UpperLimitTransitionRegionWidth=0.1  UpperLimitTransitionRegionWidthUnits=deg  PositionTargetSpecify=on  PositionTargetPriority=Low  PositionTargetValue=smiData.RevoluteJoint(44).Rz.Pos  PositionTargetValueUnits=deg  VelocityTargetSpecify=off  VelocityTargetPriority=High  VelocityTargetValue=0  VelocityTargetValueUnits=deg/s
  Tmotor_P60_Base_1_RIGID : Subsystem
  Tmotor_P60_Base_2_RIGID : Subsystem
  Tmotor_P60_Base_3_RIGID : Subsystem
  Tmotor_P60_Base_4_RIGID : Subsystem
  Tmotor_P60_Base_5_RIGID : Subsystem
  Tmotor_P60_Base_6_RIGID : Subsystem
  Tmotor_P60_Base_7_RIGID : Subsystem
  Tmotor_P60_Base_8_RIGID : Subsystem
  Tmotor_P60_Skin_1_RIGID : Subsystem
  Tmotor_P60_Skin_2_RIGID : Subsystem
  Tmotor_P60_Skin_3_RIGID : Subsystem
  Tmotor_P60_Skin_4_RIGID : Subsystem
  Tmotor_P60_Skin_5_RIGID : Subsystem
  Tmotor_P60_Skin_6_RIGID : Subsystem
  Tmotor_P60_Skin_7_RIGID : Subsystem
  Tmotor_P60_Skin_8_RIGID : Subsystem
  cw : Gain
  cw1 : Gain
  cw2 : Gain  Gain=-1
  cw3 : Gain
  rpm to deg/s : Gain  Gain=-6
  "rpm to deg/s " : Gain  Gain=-6
  "rpm to deg/s  " : Gain  Gain=6
  rpm to deg/s 1 : Gain  Gain=-6
  rpm to deg/s1 : Gain  Gain=6
  rpm to deg/s2 : Gain  Gain=6
  rpm to deg/s3 : Gain  Gain=6
  rpm to deg/s4 : Gain  Gain=-6
  F : PMIOPort  Side=Left
  F1 : PMIOPort  Port=2  Side=Left
  F2 : PMIOPort  Port=3  Side=Left
  F3 : PMIOPort  Port=4  Side=Left
  F4 : PMIOPort  Port=5  Side=Left
  F5 : PMIOPort  Port=6  Side=Left
  F6 : PMIOPort  Port=7  Side=Left
  F7 : PMIOPort  Port=8  Side=Left
  Motors Rotation [deg] : Outport
  M8 RPM : Outport  Port=2
  M7 RPM : Outport  Port=3
  M6 RPM : Outport  Port=4
  M5 RPM : Outport  Port=5
  M4 RPM : Outport  Port=6
  M3 RPM : Outport  Port=7
  M2 RPM : Outport  Port=8
  M1 RPM : Outport  Port=9
  wires:
  Thrust M8/1 -> Tmotor_P60_Base_1_RIGID/1(Thrust M8)
  Torque M8/1 -> Tmotor_P60_Base_1_RIGID/2(Torque M8)
  M8 RPM Command/1 -> "rpm to deg/s "/1
  "rpm to deg/s "/1 -> M8 TF/1(In1)
  Torque M4/1 -> Tmotor_P60_Base_2_RIGID/2(Torque M4)
  Thrust M4/1 -> Tmotor_P60_Base_2_RIGID/1(Thrust M4)
  rpm to deg/s/1 -> M4 TF/1(In1)
  M4 RPM Command/1 -> rpm to deg/s/1
  M4 TF/1(M4 RPM) -> Abs5/1
  M8 TF/1(M8 RPM) -> Abs4/1
  M1 TF/1(M1 RPM) -> Abs2/1
  M1 RPM Command/1 -> cw1/1
  "rpm to deg/s  "/1 -> M1 TF/1(In1)
  Thrust M1/1 -> Tmotor_P60_Base_5_RIGID/1(Thrust M1)
  Torque M1/1 -> Tmotor_P60_Base_5_RIGID/2(Torque M1)
  rpm to deg/s 1/1 -> M5 TF/1(In1)
  M5 TF/1(M5 RPM) -> Abs3/1
  M5 RPM Command/1 -> cw/1
  Thrust M5/1 -> Tmotor_P60_Base_3_RIGID/1(Thrust M5)
  Torque M5/1 -> Tmotor_P60_Base_3_RIGID/2(Torque M5)
  M2 TF/1(M2 RPM) -> Abs1/1
  M6 RPM Command/1 -> rpm to deg/s1/1
  rpm to deg/s1/1 -> M2 TF/1(In1)
  Thrust M6/1 -> Tmotor_P60_Base_7_RIGID/1(Thrust M2)
  Torque M6/1 -> Tmotor_P60_Base_7_RIGID/2(Torque M2)
  rpm to deg/s2/1 -> M3 TF/1(In1)
  M7 RPM Command/1 -> cw2/1
  M3 TF/1(M3 RPM) -> Abs7/1
  Torque M7/1 -> Tmotor_P60_Base_4_RIGID/2(Torque M3)
  Thrust M7/1 -> Tmotor_P60_Base_4_RIGID/1(Thrust M3)
  M7 TF/1(M7 RPM) -> Abs6/1
  M3 RPM Command/1 -> cw3/1
  rpm to deg/s3/1 -> M7 TF/1(In1)
  Torque M3/1 -> Tmotor_P60_Base_8_RIGID/2(Torque M7)
  Thrust M3/1 -> Tmotor_P60_Base_8_RIGID/1(Thrust M7)
  rpm to deg/s4/1 -> M6 TF/1(In1)
  M2 RPM Command/1 -> rpm to deg/s4/1
  M6 TF/1(M6 RPM) -> Abs/1
  Torque M2/1 -> Tmotor_P60_Base_6_RIGID/2(Torque M6)
  Thrust M2/1 -> Tmotor_P60_Base_6_RIGID/1(Thrust M6)
  cw/1 -> rpm to deg/s 1/1
  cw1/1 -> "rpm to deg/s  "/1
  cw2/1 -> rpm to deg/s2/1
  cw3/1 -> rpm to deg/s3/1
  M1 TF/2(M1 rot [deg]) -> Mux/1
  M2 TF/2(M2 rot [deg]) -> Mux/2
  M3 TF/2(M3 rot [deg]) -> Mux/3
  M4 TF/2(M4 rot [deg]) -> Mux/4
  M5 TF/2(M5 rot [de]) -> Mux/5
  M6 TF/2(M6 rot [deg]) -> Mux/6
  M7 TF/2(M7 rot [deg]) -> Mux/7
  M8 TF/2(M8 rot [deg]) -> Mux/8
  Mux/1 -> Motors Rotation [deg]/1
  Abs/1 -> M2 RPM/1
  Abs1/1 -> M6 RPM/1
  Abs2/1 -> M1 RPM/1
  Abs3/1 -> M5 RPM/1
  Abs4/1 -> M8 RPM/1
  Abs5/1 -> M4 RPM/1
  Abs6/1 -> M3 RPM/1
  Abs7/1 -> M7 RPM/1
  connections:
  Tmotor_P60_Skin_5_RIGID/RConn1 -- Prop_22_66_CCW_10_RIGID/LConn1
  F5/RConn1 -- Tmotor_P60_Base_3_RIGID/LConn1
  Revolute31/LConn1 -- Tmotor_P60_Base_2_RIGID/RConn1
  Prop_22_66_CW_7_RIGID/LConn1 -- Prop_22_66_CW_8_RIGID/LConn2
  Revolute35/LConn1 -- Tmotor_P60_Base_4_RIGID/RConn1
  Revolute37/LConn1 -- Tmotor_P60_Base_5_RIGID/RConn1
  Prop_22_66_CW_3_RIGID/RConn1 -- Prop_22_66_CW_4_RIGID/LConn2
  Prop_22_66_CW_6_RIGID/LConn1 -- Tmotor_P60_Skin_8_RIGID/RConn1
  Tmotor_P60_Skin_6_RIGID/RConn1 -- Prop_22_66_CCW_9_RIGID/LConn1
  Revolute31/RConn1 -- Tmotor_P60_Skin_2_RIGID/LConn1
  Revolute29/LConn1 -- Tmotor_P60_Base_1_RIGID/RConn1
  Revolute41/LConn1 -- Tmotor_P60_Base_7_RIGID/RConn1
  Revolute39/RConn1 -- Tmotor_P60_Skin_6_RIGID/LConn1
  Revolute33/LConn1 -- Tmotor_P60_Base_3_RIGID/RConn1
  F/RConn1 -- Tmotor_P60_Base_8_RIGID/LConn1
  Revolute37/RConn1 -- Tmotor_P60_Skin_8_RIGID/LConn1
  Revolute41/RConn1 -- Tmotor_P60_Skin_5_RIGID/LConn1
  Revolute39/LConn1 -- Tmotor_P60_Base_6_RIGID/RConn1
  Revolute43/RConn1 -- Tmotor_P60_Skin_7_RIGID/LConn1
  F1/RConn1 -- Tmotor_P60_Base_4_RIGID/LConn1
  Prop_22_66_CCW_2_RIGID/LConn1 -- Tmotor_P60_Skin_1_RIGID/RConn1
  Prop_22_66_CCW_4_RIGID/LConn1 -- Prop_22_66_CCW_3_RIGID/RConn1 -- Tmotor_P60_Skin_2_RIGID/RConn1
  Prop_22_66_CCW_10_RIGID/LConn2 -- Prop_22_66_CCW_8_RIGID/LConn1
  Prop_22_66_CCW_2_RIGID1/LConn1 -- Tmotor_P60_Skin_1_RIGID/LConn1
  Prop_22_66_CCW_7_RIGID/LConn1 -- Prop_22_66_CCW_9_RIGID/LConn2
  Revolute43/LConn1 -- Tmotor_P60_Base_8_RIGID/RConn1
  Prop_22_66_CW_1_RIGID/LConn1 -- Tmotor_P60_Skin_3_RIGID/RConn1
  Prop_22_66_CW_8_RIGID/LConn1 -- Tmotor_P60_Skin_7_RIGID/RConn1
  Revolute33/RConn1 -- Tmotor_P60_Skin_3_RIGID/LConn1
  Prop_22_66_CW_2_RIGID/LConn1 -- Prop_22_66_CW_1_RIGID/RConn1
  Prop_22_66_CW_4_RIGID/LConn1 -- Tmotor_P60_Skin_4_RIGID/RConn1
  Prop_22_66_CW_5_RIGID/LConn1 -- Tmotor_P60_Skin_8_RIGID/RConn2
  F7/RConn1 -- Tmotor_P60_Base_1_RIGID/LConn1
  Revolute35/RConn1 -- Tmotor_P60_Skin_4_RIGID/LConn1
  Revolute29/RConn1 -- Tmotor_P60_Skin_1_RIGID/LConn2
  F6/RConn1 -- Tmotor_P60_Base_2_RIGID/LConn1
  F4/RConn1 -- Tmotor_P60_Base_5_RIGID/LConn1
  F2/RConn1 -- Tmotor_P60_Base_7_RIGID/LConn1
  F3/RConn1 -- Tmotor_P60_Base_6_RIGID/LConn1
  Revolute29/LConn2 -- M8 TF/RConn1
  M4 TF/RConn1 -- Revolute31/LConn2
  Revolute37/LConn2 -- M1 TF/RConn1
  M5 TF/RConn1 -- Revolute33/LConn2
  M2 TF/RConn1 -- Revolute41/LConn2
  M3 TF/RConn1 -- Revolute35/LConn2
  M7 TF/RConn1 -- Revolute43/LConn2
  M6 TF/RConn1 -- Revolute39/LConn2

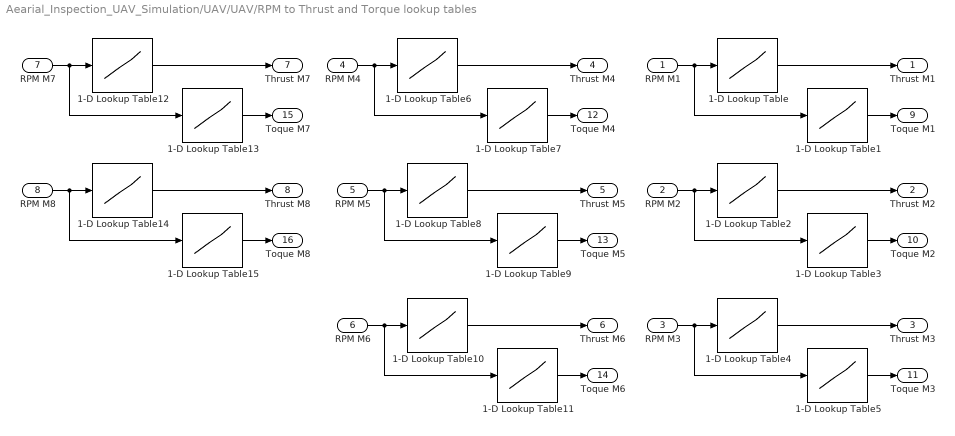
== system Aearial_Inspection_UAV_Simulation/UAV/UAV/RPM to Thrust and Torque lookup tables ==
  RPM M1 : Inport
  RPM M2 : Inport  Port=2
  RPM M3 : Inport  Port=3
  RPM M4 : Inport  Port=4
  RPM M5 : Inport  Port=5
  RPM M6 : Inport  Port=6
  RPM M7 : Inport  Port=7
  RPM M8 : Inport  Port=8
  1-D Lookup Table{,2,4,6,8,10,12,14} (8 alike) : Lookup_n-D  NumberOfTableDimensions=1  BreakpointsForDimension1=[0;Motor_data.RPM]  BeginIndexSearchUsingPreviousIndexResult=on  Table=[0;Motor_data.Thrust]  InterpMethod=Cubic spline  ExtrapMethod=Cubic spline  InternalRulePriority=Speed  RndMeth=Simplest
  1-D Lookup Table{1,3,5,7,9,11,13,15} (8 alike) : Lookup_n-D  NumberOfTableDimensions=1  BreakpointsForDimension1=[0;Motor_data.RPM]  BeginIndexSearchUsingPreviousIndexResult=on  Table=[0;Motor_data.Torque]  InterpMethod=Cubic spline  ExtrapMethod=Cubic spline  InternalRulePriority=Speed  RndMeth=Simplest
  Thrust M1 : Outport
  Thrust M2 : Outport  Port=2
  Thrust M3 : Outport  Port=3
  Thrust M4 : Outport  Port=4
  Thrust M5 : Outport  Port=5
  Thrust M6 : Outport  Port=6
  Thrust M7 : Outport  Port=7
  Thrust M8 : Outport  Port=8
  Toque M1 : Outport  Port=9
  Toque M2 : Outport  Port=10
  Toque M3 : Outport  Port=11
  Toque M4 : Outport  Port=12
  Toque M5 : Outport  Port=13
  Toque M6 : Outport  Port=14
  Toque M7 : Outport  Port=15
  Toque M8 : Outport  Port=16
  wires:
  RPM M1/1 -> 1-D Lookup Table1/1, 1-D Lookup Table/1
  1-D Lookup Table/1 -> Thrust M1/1
  1-D Lookup Table1/1 -> Toque M1/1
  1-D Lookup Table3/1 -> Toque M2/1
  1-D Lookup Table2/1 -> Thrust M2/1
  RPM M2/1 -> 1-D Lookup Table2/1, 1-D Lookup Table3/1
  RPM M3/1 -> 1-D Lookup Table5/1, 1-D Lookup Table4/1
  1-D Lookup Table4/1 -> Thrust M3/1
  1-D Lookup Table5/1 -> Toque M3/1
  1-D Lookup Table7/1 -> Toque M4/1
  1-D Lookup Table6/1 -> Thrust M4/1
  RPM M4/1 -> 1-D Lookup Table6/1, 1-D Lookup Table7/1
  RPM M5/1 -> 1-D Lookup Table9/1, 1-D Lookup Table8/1
  1-D Lookup Table8/1 -> Thrust M5/1
  1-D Lookup Table9/1 -> Toque M5/1
  1-D Lookup Table11/1 -> Toque M6/1
  1-D Lookup Table10/1 -> Thrust M6/1
  RPM M6/1 -> 1-D Lookup Table10/1, 1-D Lookup Table11/1
  RPM M7/1 -> 1-D Lookup Table13/1, 1-D Lookup Table12/1
  1-D Lookup Table12/1 -> Thrust M7/1
  1-D Lookup Table13/1 -> Toque M7/1
  1-D Lookup Table15/1 -> Toque M8/1
  1-D Lookup Table14/1 -> Thrust M8/1
  RPM M8/1 -> 1-D Lookup Table14/1, 1-D Lookup Table15/1

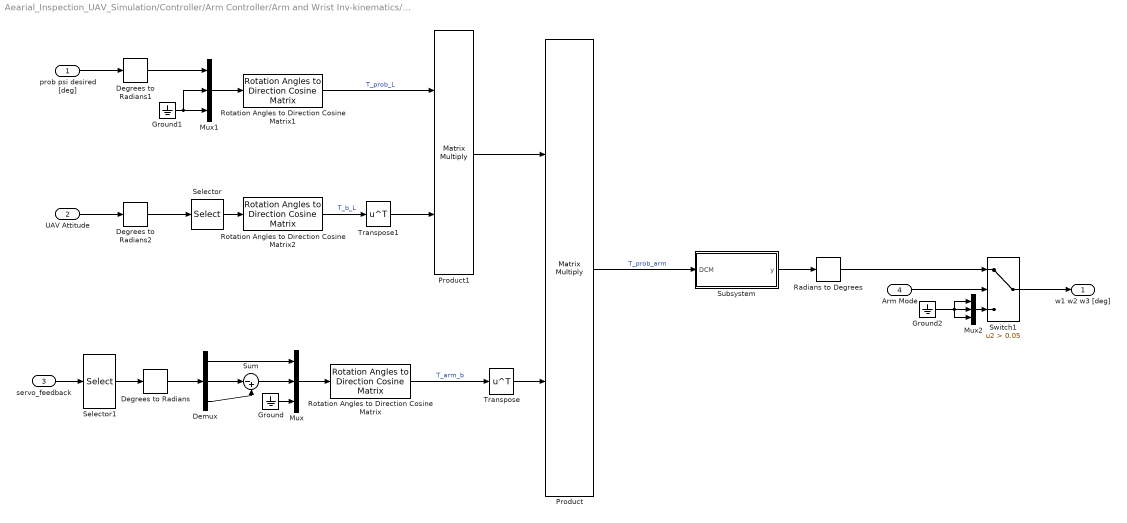
== system Aearial_Inspection_UAV_Simulation/Controller/Arm Controller/Arm and Wrist Inv-kinematics/wrist Controller ==
  prob psi desired [deg] : Inport
  UAV Attitude : Inport  Port=2
  servo_feedback : Inport  Port=3
  Arm Mode : Inport  Port=4
  Degrees to Radians : simulink_extras/Transformations/Degrees to Radians
  Degrees to Radians1 : simulink_extras/Transformations/Degrees to Radians
  Degrees to Radians2 : simulink_extras/Transformations/Degrees to Radians
  Demux : Demux  Outputs=3
  Ground : Ground
  Ground1 : Ground
  Ground2 : Ground
  Mux : Mux  Inputs=3
  Mux1 : Mux  Inputs=3
  Mux2 : Mux  Inputs=3
  Product : Product  Multiplication=Matrix(*)
  Product1 : Product  Multiplication=Matrix(*)
  Radians to Degrees : simulink_extras/Transformations/Radians to Degrees
  Rotation Angles to Direction Cosine Matrix : sharedtransform/Rotation Angles to Direction Cosine Matrix  rotationOrder=ZYX  aMode=aMode
  Rotation Angles to Direction Cosine Matrix1 : sharedtransform/Rotation Angles to Direction Cosine Matrix  rotationOrder=ZYX  aMode=aMode
  Rotation Angles to Direction Cosine Matrix2 : sharedtransform/Rotation Angles to Direction Cosine Matrix  rotationOrder=ZYX  aMode=aMode
  Selector : Selector  InputPortWidth=3  IndexOptions=Index vector (dialog)  Indices=[3 2 1]  OutputSizes=1
  Selector1 : Selector  InputPortWidth=6  IndexOptions=Index vector (dialog)  Indices=1:3  OutputSizes=1
  Subsystem : Subsystem
  Sum : Sum  Inputs=|-+
  Switch1 : Switch  Criteria=u2 > Threshold  Threshold=0.05  SaturateOnIntegerOverflow=off  InputSameDT=off
  Transpose : Math  Operator=transpose
  Transpose1 : Math  Operator=transpose
  w1 w2 w3 [deg] : Outport  PortDimensions=3
  wires:
  Demux/2 -> Sum/1
  Demux/3 -> Sum/2
  Sum/1 -> Mux/2
  Demux/1 -> Mux/1
  Ground/1 -> Mux/3
  Mux/1 -> Rotation Angles to Direction Cosine Matrix/1
  Mux1/1 -> Rotation Angles to Direction Cosine Matrix1/1
  Degrees to Radians/1 -> Demux/1
  prob psi desired [deg]/1 -> Degrees to Radians1/1
  Degrees to Radians1/1 -> Mux1/1
  Ground1/1 -> Mux1/2, Mux1/3
  Rotation Angles to Direction Cosine Matrix/1 -> Transpose/1  "T_arm_b"
  Subsystem/1(y) -> Radians to Degrees/1
  Rotation Angles to Direction Cosine Matrix2/1 -> Transpose1/1  "T_b_L"
  Product/1 -> Subsystem/1(DCM)  "T_prob_arm"
  Radians to Degrees/1 -> Switch1/1
  UAV Attitude/1 -> Degrees to Radians2/1
  Selector/1 -> Rotation Angles to Direction Cosine Matrix2/1
  Rotation Angles to Direction Cosine Matrix1/1 -> Product1/1  "T_prob_L"
  Product1/1 -> Product/1
  Degrees to Radians2/1 -> Selector/1
  Transpose1/1 -> Product1/2
  Transpose/1 -> Product/2
  Mux2/1 -> Switch1/3
  Arm Mode/1 -> Switch1/2
  servo_feedback/1 -> Selector1/1
  Ground2/1 -> Mux2/2, Mux2/3, Mux2/1
  Switch1/1 -> w1 w2 w3 [deg]/1
  Selector1/1 -> Degrees to Radians/1

== system Aearial_Inspection_UAV_Simulation/Controller/UAV Controller/      1/      ==
  phi_d theta_d psi_d : Inport
  Demux : Demux  Outputs=3
  Gain : Gain  Gain=Btheta  Multiplication=Matrix(K*u)
  Gain1 : Gain  Gain=Atheta  Multiplication=Matrix(K*u)
  Gain2 : Gain  Gain=Bphi  Multiplication=Matrix(K*u)
  Gain3 : Gain  Gain=Aphi  Multiplication=Matrix(K*u)
  Gain4 : Gain  Gain=Bpsi  Multiplication=Matrix(K*u)
  Gain5 : Gain  Gain=Apsi  Multiplication=Matrix(K*u)
  Ground : Ground
  Integrator : Integrator
  Integrator1 : Integrator
  Integrator2 : Integrator
  Mux : Mux  Inputs=3
  Sum : Sum  Inputs=|++
  Sum1 : Sum  Inputs=|++
  Sum2 : Sum  Inputs=|++
  Terminator : Terminator
  "[phi_d, phi_d_dot] [theta_d, theta_d_dot] [psi_d, psi_d_dot]" : Outport
  wires:
  phi_d theta_d psi_d/1 -> Terminator/1
  Gain/1 -> Sum/1
  Sum/1 -> Integrator/1
  Gain1/1 -> Sum/2
  Integrator/1 -> Gain1/1, Mux/2  "[theta_d, theta_d_dot]"
  Mux/1 -> "[phi_d, phi_d_dot] [theta_d, theta_d_dot] [psi_d, psi_d_dot]"/1
  Integrator1/1 -> Gain3/1, Mux/1  "[phi_d, phi_d_dot]"
  Gain3/1 -> Sum1/2
  Sum1/1 -> Integrator1/1
  Gain2/1 -> Sum1/1
  Demux/1 -> Gain2/1  "phi_d"
  Demux/2 -> Gain/1  "theta_d"
  Demux/3 -> Gain4/1  "psi_d"
  Integrator2/1 -> Gain5/1, Mux/3  "[psi_d, psi_d_dot]"
  Gain5/1 -> Sum2/2
  Sum2/1 -> Integrator2/1
  Gain4/1 -> Sum2/1
  Ground/1 -> Demux/1
